simulink model "Full_model"  (R2020a)
settings: Solver=VariableStepAuto  StartTime=0.0  StopTime=1  FixedStep=0.0001  MaxStep=0.001  RelTol=1e-3  EnableMultiTasking=on
values from neighbouring files (symbols this model uses):
  motor_diamter = 25/1000    (= 0.025)    [parameters.m]
  motor_height = 56/1000    (= 0.056)    [parameters.m]
  pulley_diameterOut = 1/100    (= 0.01)    [parameters.m]
undefined symbols (not defined in the file or in its folder): Local, X, Y, Z
libraries: sm_lib x59, Multibody_Parts_Lib x22, nesl_utility x5
(part 2 of 2)

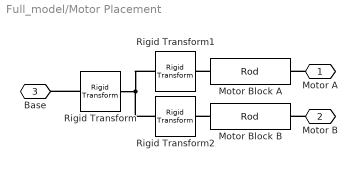
== system Full_model/Motor Placement ==
  Motor Block A : Multibody_Parts_Lib/Basic/Rod  rod_rad=motor_diamter/2  rod_len=motor_height  rod_rho=7000  rod_color=motor_colA  rod_opc=1  popup_zori=Local +Z  popup_markings=None  mark_radius_range=[0.5 1.01]  mark_length_range=1.005  mark_angle_range=30  mark_color=[1 1 1]
      settings: SourceProductName=Simscape Multibody Parts Library
  Motor Block B : Multibody_Parts_Lib/Basic/Rod  rod_rad=motor_diamter/2  rod_len=motor_height  rod_rho=7000  rod_color=motor_colB  rod_opc=1  popup_zori=Local +Z  popup_markings=None  mark_radius_range=[0.5 1.01]  mark_length_range=1.005  mark_angle_range=30  mark_color=[1 1 1]
      settings: SourceProductName=Simscape Multibody Parts Library
  Rigid Transform : sm_lib/Frames and Transforms/Rigid Transform  TranslationMethod=StandardAxis  TranslationStandardOffset=motorDisplacement_y  TranslationLengthUnit=m  TranslationStandardAxis=-Y  TranslationCartesianOffset=[0 0 0]  TranslationROffset=0  TranslationROffsetUnits=m  TranslationZOffset=0  TranslationZOffsetUnits=m  TranslationThetaOffset=0  TranslationThetaOffsetUnits=deg  RotationMethod=None  RotationAngleUnits=deg  RotationStandardAxis=+Z  RotationAngle=0.0  RotationArbitraryAxis=[0 0 1]  FollAlignAxisA=+X  BaseAlignAxisA=+Y  FollAlignAxisB=+Y  BaseAlignAxisB=+Z  RotationSequenceAxes=FollowerAxes  RotationSequence=XYX  RotationSequenceAngles=[0 0 0]  RotationSequenceAnglesUnits=deg  RotationMatrix=[1 0 0; 0 1 0; 0 0 1]
  Rigid Transform1 : sm_lib/Frames and Transforms/Rigid Transform  TranslationMethod=StandardAxis  TranslationStandardOffset=motorDisplacement_x  TranslationLengthUnit=m  TranslationStandardAxis=-X  TranslationCartesianOffset=[0 0 0]  TranslationROffset=0  TranslationROffsetUnits=m  TranslationZOffset=0  TranslationZOffsetUnits=m  TranslationThetaOffset=0  TranslationThetaOffsetUnits=deg  RotationMethod=StandardAxis  RotationAngleUnits=deg  RotationStandardAxis=-X  RotationAngle=0.0  RotationArbitraryAxis=[0 0 1]  FollAlignAxisA=+X  BaseAlignAxisA=+Y  FollAlignAxisB=+Y  BaseAlignAxisB=+Z  RotationSequenceAxes=FollowerAxes  RotationSequence=XYX  RotationSequenceAngles=[0 0 0]  RotationSequenceAnglesUnits=deg  RotationMatrix=[1 0 0; 0 1 0; 0 0 1]
  Rigid Transform2 : sm_lib/Frames and Transforms/Rigid Transform  TranslationMethod=StandardAxis  TranslationStandardOffset=motorDisplacement_x  TranslationLengthUnit=m  TranslationStandardAxis=+X  TranslationCartesianOffset=[0 0 0]  TranslationROffset=0  TranslationROffsetUnits=m  TranslationZOffset=0  TranslationZOffsetUnits=m  TranslationThetaOffset=0  TranslationThetaOffsetUnits=deg  RotationMethod=StandardAxis  RotationAngleUnits=deg  RotationStandardAxis=-X  RotationAngle=0.0  RotationArbitraryAxis=[0 0 1]  FollAlignAxisA=+X  BaseAlignAxisA=+Y  FollAlignAxisB=+Y  BaseAlignAxisB=+Z  RotationSequenceAxes=FollowerAxes  RotationSequence=XYX  RotationSequenceAngles=[0 0 0]  RotationSequenceAnglesUnits=deg  RotationMatrix=[1 0 0; 0 1 0; 0 0 1]
  Motor A : PMIOPort  Side=Right
  Motor B : PMIOPort  Port=2  Side=Right
  Base : PMIOPort  Port=3  Side=Left
  connections:
  Motor Block A/LConn1 -- Rigid Transform1/RConn1
  Motor B/RConn1 -- Motor Block B/RConn1
  Rigid Transform1/LConn1 -- Rigid Transform/RConn1 -- Rigid Transform2/LConn1
  Motor A/RConn1 -- Motor Block A/RConn1
  Rigid Transform/LConn1 -- Base/RConn1
  Motor Block B/LConn1 -- Rigid Transform2/RConn1

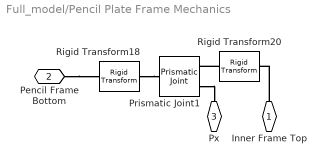
== system Full_model/Pencil Plate Frame Mechanics ==
  Prismatic Joint1 : sm_lib/Joints/Prismatic Joint  JointMode=Normal  SenseConstraintForce=off  SenseConstraintForceX=off  SenseConstraintForceY=off  SenseConstraintForceZ=off  SenseConstraintTorque=off  SenseConstraintTorqueX=off  SenseConstraintTorqueY=off  SenseConstraintTorqueZ=off  SenseTotalForce=off  SenseTotalForceX=off  SenseTotalForceY=off  SenseTotalForceZ=off  SenseTotalTorque=off  SenseTotalTorqueX=off  SenseTotalTorqueY=off  SenseTotalTorqueZ=off  CompositeWrenchDir=FollowerOnBase  CompositeWrenchFrame=BaseFrame  EquilibriumPosition=0  EquilibriumPositionUnits=m  SpringStiffness=0  SpringStiffnessUnits=N/m  DampingCoefficient=0  DampingCoefficientUnits=N/(m/s)  TorqueActuationMode=NoTorque  MotionActuationMode=ComputedMotion  SensePosition=on  SenseVelocity=off  SenseAcceleration=off  SenseTorqueForce=off  SenseLowerLimitTorqueForce=off  SenseUpperLimitTorqueForce=off  LowerLimitSpecify=on  LowerLimitBound=-0.15  LowerLimitBoundUnits=m  LowerLimitStiffness=1e6  LowerLimitStiffnessUnits=N/m  LowerLimitDamping=1e3  LowerLimitDampingUnits=N/(m/s)  LowerLimitTransitionRegionWidth=1e-4  LowerLimitTransitionRegionWidthUnits=m  UpperLimitSpecify=on  UpperLimitBound=0.15  UpperLimitBoundUnits=m  UpperLimitStiffness=1e6  UpperLimitStiffnessUnits=N/m  UpperLimitDamping=1e3  UpperLimitDampingUnits=N/(m/s)  UpperLimitTransitionRegionWidth=1e-4  UpperLimitTransitionRegionWidthUnits=m  PositionTargetSpecify=off  PositionTargetPriority=High  PositionTargetValue=0  PositionTargetValueUnits=m  VelocityTargetSpecify=off  VelocityTargetPriority=High  VelocityTargetValue=0  VelocityTargetValueUnits=m/s
  Rigid Transform18 : sm_lib/Frames and Transforms/Rigid Transform  TranslationMethod=None  TranslationStandardOffset=0.1  TranslationLengthUnit=m  TranslationStandardAxis=+Z  TranslationCartesianOffset=p_itlB  TranslationROffset=0  TranslationROffsetUnits=m  TranslationZOffset=0  TranslationZOffsetUnits=m  TranslationThetaOffset=0  TranslationThetaOffsetUnits=deg  RotationMethod=StandardAxis  RotationAngleUnits=deg  RotationStandardAxis=-Y  RotationAngle=90  RotationArbitraryAxis=[0 0 1]  FollAlignAxisA=+X  BaseAlignAxisA=+Y  FollAlignAxisB=+Y  BaseAlignAxisB=+Z  RotationSequenceAxes=FollowerAxes  RotationSequence=XYX  RotationSequenceAngles=[0 0 0]  RotationSequenceAnglesUnits=deg  RotationMatrix=[1 0 0; 0 1 0; 0 0 1]
  Rigid Transform20 : sm_lib/Frames and Transforms/Rigid Transform  TranslationMethod=None  TranslationStandardOffset=0.1  TranslationLengthUnit=m  TranslationStandardAxis=-Z  TranslationCartesianOffset=p_itlB  TranslationROffset=0  TranslationROffsetUnits=m  TranslationZOffset=0  TranslationZOffsetUnits=m  TranslationThetaOffset=0  TranslationThetaOffsetUnits=deg  RotationMethod=StandardAxis  RotationAngleUnits=deg  RotationStandardAxis=+Y  RotationAngle=90  RotationArbitraryAxis=[0 0 1]  FollAlignAxisA=+X  BaseAlignAxisA=+Y  FollAlignAxisB=+Y  BaseAlignAxisB=+Z  RotationSequenceAxes=FollowerAxes  RotationSequence=XYX  RotationSequenceAngles=[0 0 0]  RotationSequenceAnglesUnits=deg  RotationMatrix=[1 0 0; 0 1 0; 0 0 1]
  Inner Frame Top : PMIOPort  Side=Right
  Pencil Frame Bottom : PMIOPort  Port=2  Side=Right
  Px : PMIOPort  Port=3  Side=Right
  connections:
  Rigid Transform18/RConn1 -- Prismatic Joint1/LConn1
  Rigid Transform20/LConn1 -- Prismatic Joint1/RConn1
  Prismatic Joint1/RConn2 -- Px/RConn1
  Inner Frame Top/RConn1 -- Rigid Transform20/RConn1
  Pencil Frame Bottom/RConn1 -- Rigid Transform18/LConn1

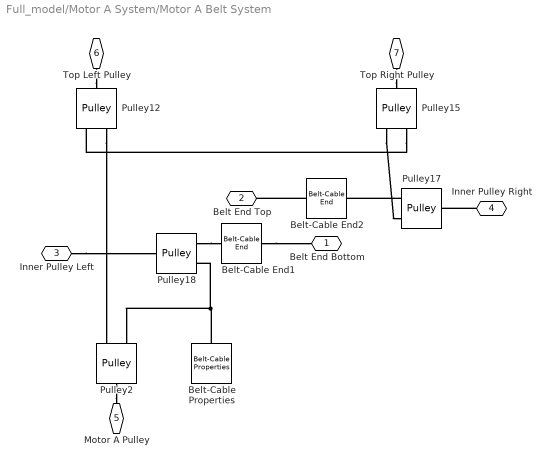
== system Full_model/Motor A System/Motor A Belt System ==
  Belt-Cable Properties : sm_lib/Belts and Cables/Belt-Cable Properties  DrumBeltCableAlignment=Unrestricted  GraphicType=PitchLine  GraphicVisPropType=SimpleVisualProperties  GraphicDiffuseColor=motor_colA  GraphicSpecularColor=[0.5 0.5 0.5 1.0]  GraphicAmbientColor=[0.15 0.15 0.15 1.0]  GraphicEmissiveColor=[0.0 0.0 0.0 1.0]  GraphicShininess=75  GraphicOpacity=1.0
      settings: SourceProductBaseCode=MS
  Belt-Cable End1 : sm_lib/Belts and Cables/Belt-Cable End
      settings: SourceProductBaseCode=MS
  Belt-Cable End2 : sm_lib/Belts and Cables/Belt-Cable End
      settings: SourceProductBaseCode=MS
  Pulley{2,12,15,17..18} (5 alike) : sm_lib/Belts and Cables/Pulley  PitchRadius=5  PitchRadiusUnits=mm  InitialWrapAngleLowerBound=0.0  InitialWrapAngleLowerBoundUnits=deg  SenseWrapAngle=off  SensePulleyAngleA=off  SensePulleyAngleB=off  SenseFleetAngleA=off  SenseFleetAngleB=off
      settings: SourceProductBaseCode=MS
  Belt End Bottom : PMIOPort  Side=Left
  Belt End Top : PMIOPort  Port=2  Side=Left
  Inner Pulley Left : PMIOPort  Port=3  Side=Left
  Inner Pulley Right : PMIOPort  Port=4  Side=Left
  Motor A Pulley : PMIOPort  Port=5  Side=Left
  Top Left Pulley : PMIOPort  Port=6  Side=Left
  Top Right Pulley : PMIOPort  Port=7  Side=Left
  connections:
  Pulley18/RConn1 -- Belt-Cable End1/RConn1
  Pulley12/RConn2 -- Pulley2/RConn1
  Belt-Cable Properties/LConn1 -- Pulley18/RConn2 -- Pulley2/RConn2
  Top Right Pulley/RConn1 -- Pulley15/LConn1
  Pulley15/RConn2 -- Pulley12/RConn1
  Pulley2/LConn1 -- Motor A Pulley/RConn1
  Top Left Pulley/RConn1 -- Pulley12/LConn1
  Belt-Cable End2/LConn1 -- Belt End Top/RConn1
  Belt-Cable End1/LConn1 -- Belt End Bottom/RConn1
  Inner Pulley Right/RConn1 -- Pulley17/LConn1
  Inner Pulley Left/RConn1 -- Pulley18/LConn1
  Pulley15/RConn1 -- Pulley17/RConn2
  Pulley17/RConn1 -- Belt-Cable End2/RConn1

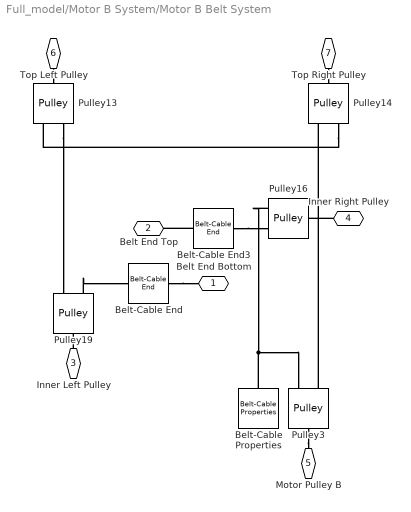
== system Full_model/Motor B System/Motor B Belt System ==
  Belt-Cable Properties : sm_lib/Belts and Cables/Belt-Cable Properties  DrumBeltCableAlignment=Unrestricted  GraphicType=PitchLine  GraphicVisPropType=SimpleVisualProperties  GraphicDiffuseColor=motor_colB  GraphicSpecularColor=[0.5 0.5 0.5 1.0]  GraphicAmbientColor=[0.15 0.15 0.15 1.0]  GraphicEmissiveColor=[0.0 0.0 0.0 1.0]  GraphicShininess=75  GraphicOpacity=1.0
      settings: SourceProductBaseCode=MS
  Belt-Cable End : sm_lib/Belts and Cables/Belt-Cable End
      settings: SourceProductBaseCode=MS
  Belt-Cable End3 : sm_lib/Belts and Cables/Belt-Cable End
      settings: SourceProductBaseCode=MS
  Pulley{3,13..14,16,19} (5 alike) : sm_lib/Belts and Cables/Pulley  PitchRadius=5  PitchRadiusUnits=mm  InitialWrapAngleLowerBound=0.0  InitialWrapAngleLowerBoundUnits=deg  SenseWrapAngle=off  SensePulleyAngleA=off  SensePulleyAngleB=off  SenseFleetAngleA=off  SenseFleetAngleB=off
      settings: SourceProductBaseCode=MS
  Belt End Bottom : PMIOPort  Side=Left
  Belt End Top : PMIOPort  Port=2  Side=Left
  Inner Left Pulley : PMIOPort  Port=3  Side=Left
  Inner Right Pulley : PMIOPort  Port=4  Side=Left
  Motor Pulley B : PMIOPort  Port=5  Side=Left
  Top Left Pulley : PMIOPort  Port=6  Side=Left
  Top Right Pulley : PMIOPort  Port=7  Side=Left
  connections:
  Inner Right Pulley/RConn1 -- Pulley16/LConn1
  Pulley19/RConn2 -- Belt-Cable End/RConn1
  Pulley14/RConn2 -- Pulley13/RConn1
  Pulley3/LConn1 -- Motor Pulley B/RConn1
  Pulley3/RConn2 -- Pulley14/RConn1
  Belt-Cable Properties/LConn1 -- Pulley3/RConn1 -- Pulley16/RConn1
  Belt-Cable End/LConn1 -- Belt End Bottom/RConn1
  Pulley13/RConn2 -- Pulley19/RConn1
  Inner Left Pulley/RConn1 -- Pulley19/LConn1
  Belt-Cable End3/LConn1 -- Belt End Top/RConn1
  Top Right Pulley/RConn1 -- Pulley14/LConn1
  Top Left Pulley/RConn1 -- Pulley13/LConn1
  Belt-Cable End3/RConn1 -- Pulley16/RConn2
